simulink model "templateLCO"  (R2023a)
settings: Solver=VariableStepAuto  StartTime=0.0  StopTime=100  FixedStep=0.00001  MaxStep=0.001  RelTol=1e-5
undefined symbols (not defined in the file): A, B0, B1, B2, Ca, constantAeroForce, constantStruForce, D0, D1, D2, invMC, invMK, lref, Mhh, nAero, nStru, options, qInitial, rho, Ugap
libraries: cstblocks x1
settings Model: Creator=Nicola Fonzi  LastModifiedBy=nicol
settings SolverCC: ZeroCrossAlgorithm=Adaptive  AlgebraicLoopSolver=TrustRegion
settings DebuggingCC: UnconnectedInputMsg=warning  UnconnectedOutputMsg=warning  UnconnectedLineMsg=warning
settings ModelReferenceCC: EnableRefExpFcnMdlSchedulingChecks=on
settings RTWCC: DLArmComputeVersion=19.05

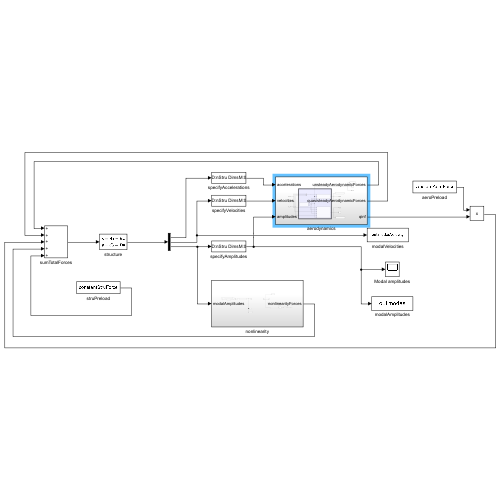
[thumbnail: Simulink's stored preview of the top-level diagram]
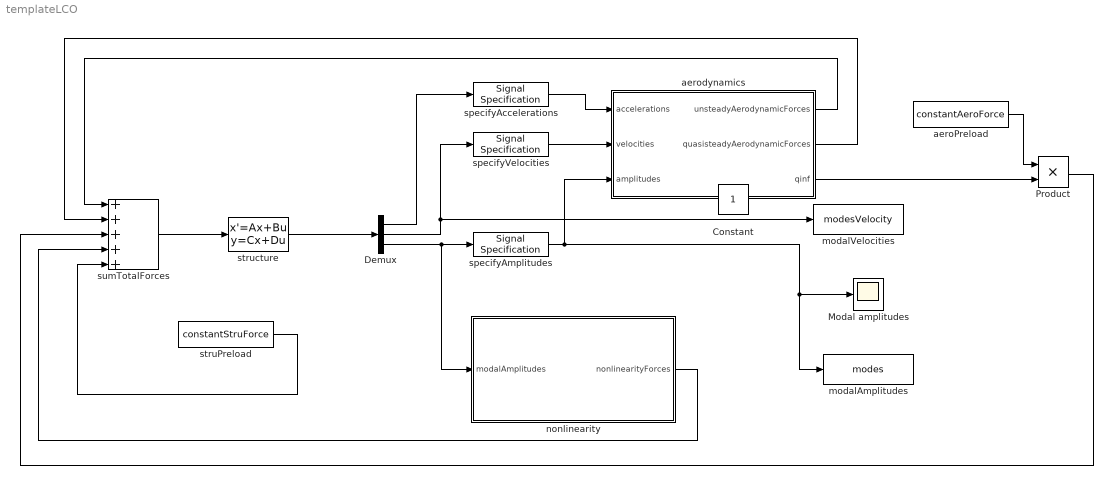
== system templateLCO ==
  Demux : Demux  Outputs=3
  Modal amplitudes : Scope
  Product : Product
  aeroPreload : Constant  Value=constantAeroForce
  aerodynamics : Subsystem
  modalAmplitudes : ToWorkspace  VariableName=modes  SaveFormat=Structure  SampleTime=-1
      settings: Save2DSignal=2-D array (concatenate along first dimension)
  modalVelocities : ToWorkspace  VariableName=modesVelocity  SaveFormat=Structure  SampleTime=-1
      settings: MaxDataPoints=1  Save2DSignal=2-D array (concatenate along first dimension)
  nonlinearity : Subsystem
  specifyAccelerations : SignalSpecification  Dimensions=nStru
  specifyAmplitudes : SignalSpecification  Dimensions=nStru
  specifyVelocities : SignalSpecification  Dimensions=nStru
  struPreload : Constant  Value=constantStruForce
  structure : StateSpace  A=[-invMC -invMK; eye(nStru) zeros(nStru)]  B=[inv(Mhh);zeros(nStru)]  C=[-invMC -invMK;eye(nStru) zeros(nStru);zeros(nStru) eye(nStru)]  D=[inv(Mhh);zeros(nStru);zeros(nStru)]  InitialCondition=qInitial
  sumTotalForces : Sum  Inputs=+++++
  Constant : Constant  IOType=siggen
  wires:
  structure/1 -> Demux/1
  sumTotalForces/1 -> structure/1
  Demux/3 -> nonlinearity/1(modalAmplitudes), specifyAmplitudes/1
  Demux/1 -> specifyAccelerations/1
  Demux/2 -> specifyVelocities/1, modalVelocities/1
  aerodynamics/1(unsteadyAerodynamicForces) -> sumTotalForces/1
  aerodynamics/2(quasisteadyAerodynamicForces) -> sumTotalForces/2
  specifyAccelerations/1 -> aerodynamics/1(accelerations)
  specifyVelocities/1 -> aerodynamics/2(velocities)
  specifyAmplitudes/1 -> modalAmplitudes/1, Modal amplitudes/1, aerodynamics/3(amplitudes)
  aerodynamics/3(qinf) -> Product/2
  aeroPreload/1 -> Product/1
  Product/1 -> sumTotalForces/3
  nonlinearity/1(nonlinearityForces) -> sumTotalForces/4
  struPreload/1 -> sumTotalForces/5

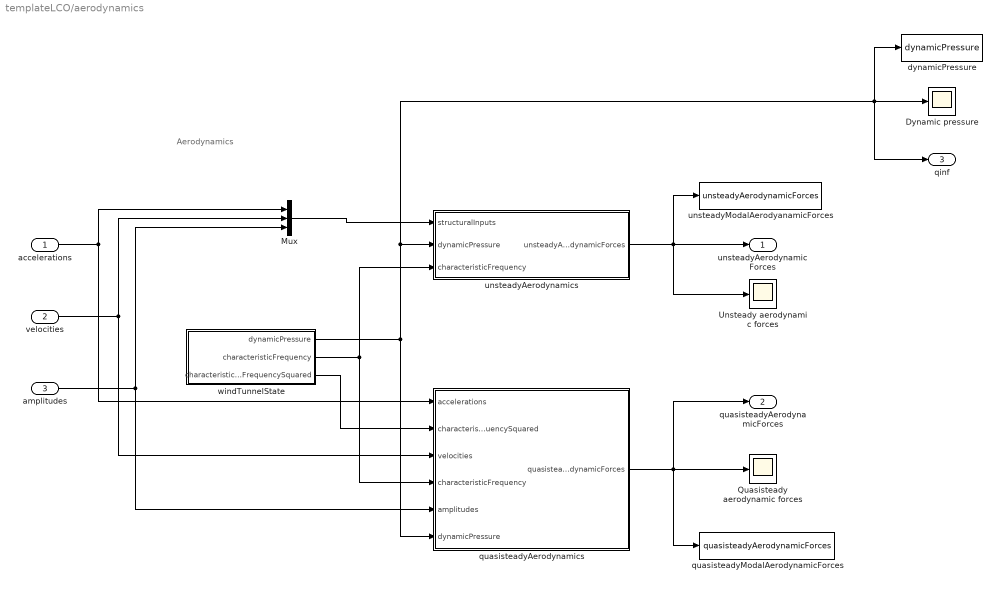
== system templateLCO/aerodynamics ==
  note: Aerodynamics
  accelerations : Inport
  velocities : Inport  Port=2
  amplitudes : Inport  Port=3
  Dynamic pressure : Scope
  Mux : Mux  Inputs=3
  Quasisteady aerodynamic forces : Scope
  Unsteady aerodynamic forces : Scope
  dynamicPressure : ToWorkspace  VariableName=dynamicPressure  SaveFormat=Structure  SampleTime=-1
      settings: Save2DSignal=2-D array (concatenate along first dimension)
  quasisteadyAerodynamics : Subsystem
  quasisteadyModalAerodynamicForces : ToWorkspace  VariableName=quasisteadyAerodynamicForces  SaveFormat=Structure  SampleTime=-1
      settings: Save2DSignal=2-D array (concatenate along first dimension)
  unsteadyAerodynamics : Subsystem
  unsteadyModalAerodyanamicForces : ToWorkspace  VariableName=unsteadyAerodynamicForces  SaveFormat=Structure  SampleTime=-1
      settings: Save2DSignal=2-D array (concatenate along first dimension)
  windTunnelState : Subsystem
  unsteadyAerodynamicForces : Outport
  quasisteadyAerodynamicForces : Outport  Port=2
  qinf : Outport  Port=3
  wires:
  windTunnelState/1(dynamicPressure) -> qinf/1, dynamicPressure/1, Dynamic pressure/1, unsteadyAerodynamics/2(dynamicPressure), quasisteadyAerodynamics/6(dynamicPressure)
  windTunnelState/2(characteristicFrequency) -> unsteadyAerodynamics/3(characteristicFrequency), quasisteadyAerodynamics/4(characteristicFrequency)
  windTunnelState/3(characteristicFrequencySquared) -> quasisteadyAerodynamics/2(characteristicFrequencySquared)
  accelerations/1 -> quasisteadyAerodynamics/1(accelerations), Mux/1
  velocities/1 -> quasisteadyAerodynamics/3(velocities), Mux/2
  amplitudes/1 -> quasisteadyAerodynamics/5(amplitudes), Mux/3
  Mux/1 -> unsteadyAerodynamics/1(structuralInputs)
  unsteadyAerodynamics/1(unsteadyAerodynamicForces) -> unsteadyModalAerodyanamicForces/1, Unsteady aerodynamic forces/1, unsteadyAerodynamicForces/1
  quasisteadyAerodynamics/1(quasisteadyAerodynamicForces) -> quasisteadyModalAerodynamicForces/1, quasisteadyAerodynamicForces/1, Quasisteady aerodynamic forces/1

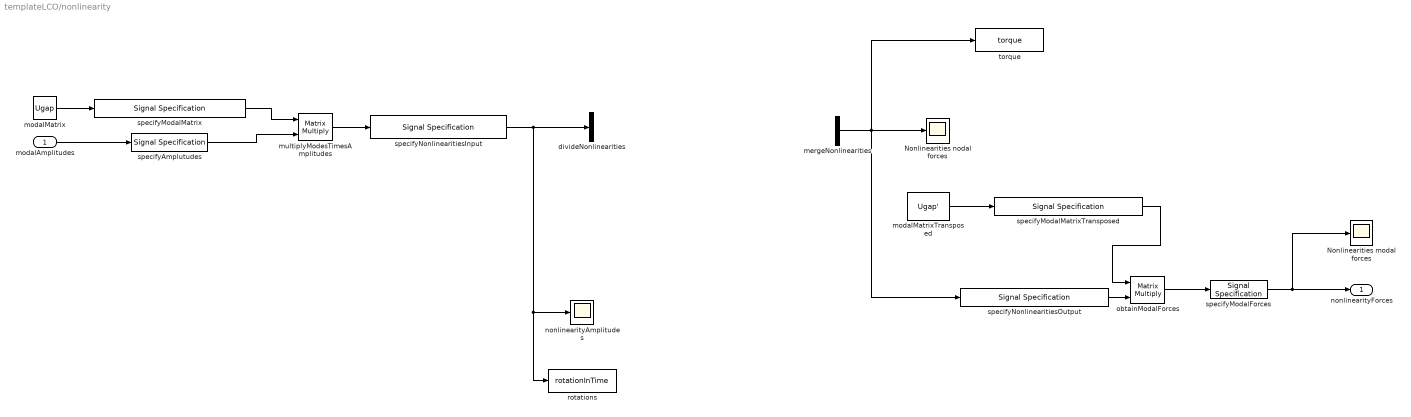
== system templateLCO/nonlinearity ==
  modalAmplitudes : Inport
  Nonlinearities modal forces : Scope
  Nonlinearities nodal forces : Scope
  divideNonlinearities : Demux  Outputs=2
  mergeNonlinearities : Mux  Inputs=2
  modalMatrix : Constant  Value=Ugap
  modalMatrixTransposed : Constant  Value=Ugap'
  multiplyModesTimesAmplitudes : Product  Multiplication=Matrix(*)
  nonlinearityAmplitudes : Scope
  obtainModalForces : Product  Multiplication=Matrix(*)
  rotations : ToWorkspace  VariableName=rotationInTime  SaveFormat=Structure With Time  SampleTime=-1
  specifyAmplutudes : SignalSpecification  Dimensions=[nStru,1]
  specifyModalForces : SignalSpecification  Dimensions=nStru
  specifyModalMatrix : SignalSpecification  Dimensions=[size(options.gapPoints,1),nStru]
  specifyModalMatrixTransposed : SignalSpecification  Dimensions=[nStru,size(options.gapPoints,1)]
  specifyNonlinearitiesInput : SignalSpecification  Dimensions=size(options.gapPoints,1)
  specifyNonlinearitiesOutput : SignalSpecification  Dimensions=[size(options.gapPoints,1),1]
  torque : ToWorkspace  VariableName=torque  SaveFormat=Structure With Time  SampleTime=-1
  nonlinearityForces : Outport
  wires:
  modalMatrixTransposed/1 -> specifyModalMatrixTransposed/1
  modalMatrix/1 -> specifyModalMatrix/1
  mergeNonlinearities/1 -> torque/1, specifyNonlinearitiesOutput/1, Nonlinearities nodal forces/1
  obtainModalForces/1 -> specifyModalForces/1
  specifyModalMatrix/1 -> multiplyModesTimesAmplitudes/1
  specifyAmplutudes/1 -> multiplyModesTimesAmplitudes/2
  modalAmplitudes/1 -> specifyAmplutudes/1
  specifyNonlinearitiesInput/1 -> divideNonlinearities/1, nonlinearityAmplitudes/1, rotations/1
  multiplyModesTimesAmplitudes/1 -> specifyNonlinearitiesInput/1
  specifyModalForces/1 -> nonlinearityForces/1, Nonlinearities modal forces/1
  specifyNonlinearitiesOutput/1 -> obtainModalForces/2
  specifyModalMatrixTransposed/1 -> obtainModalForces/1

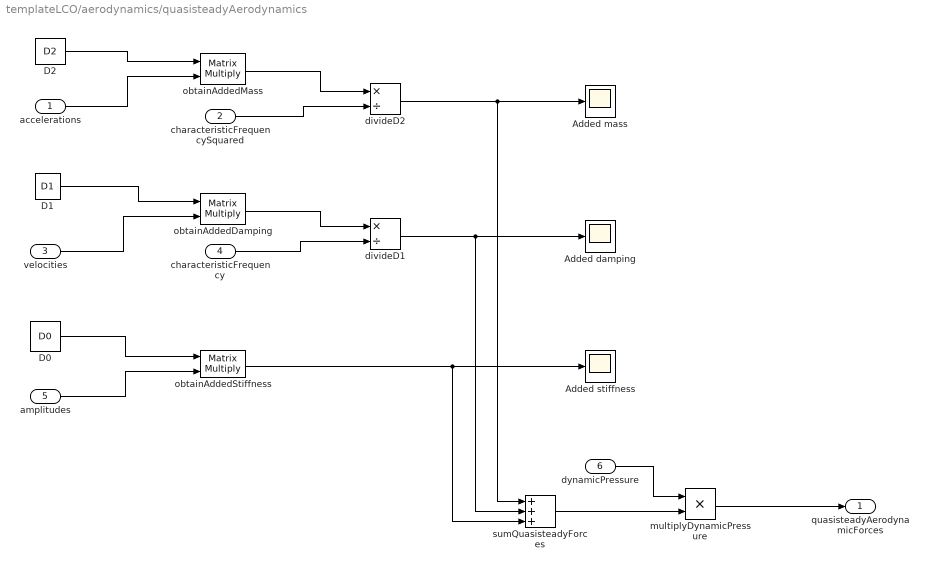
== system templateLCO/aerodynamics/quasisteadyAerodynamics ==
  accelerations : Inport
  characteristicFrequencySquared : Inport  Port=2
  velocities : Inport  Port=3
  characteristicFrequency : Inport  Port=4
  amplitudes : Inport  Port=5
  dynamicPressure : Inport  Port=6
  Added damping : Scope
  Added mass : Scope
  Added stiffness : Scope
  D0 : Constant  Value=D0
  D1 : Constant  Value=D1
  D2 : Constant  Value=D2
  divideD1 : Product  Inputs=*/
  divideD2 : Product  Inputs=*/
  multiplyDynamicPressure : Product
  obtainAddedDamping : Product  Multiplication=Matrix(*)
  obtainAddedMass : Product  Multiplication=Matrix(*)
  obtainAddedStiffness : Product  Multiplication=Matrix(*)
  sumQuasisteadyForces : Sum  Inputs=+++
  quasisteadyAerodynamicForces : Outport
  wires:
  amplitudes/1 -> obtainAddedStiffness/2
  obtainAddedDamping/1 -> divideD1/1
  divideD2/1 -> Added mass/1, sumQuasisteadyForces/1
  sumQuasisteadyForces/1 -> multiplyDynamicPressure/2
  dynamicPressure/1 -> multiplyDynamicPressure/1
  D2/1 -> obtainAddedMass/1
  divideD1/1 -> sumQuasisteadyForces/2, Added damping/1
  obtainAddedMass/1 -> divideD2/1
  D1/1 -> obtainAddedDamping/1
  obtainAddedStiffness/1 -> sumQuasisteadyForces/3, Added stiffness/1
  D0/1 -> obtainAddedStiffness/1
  velocities/1 -> obtainAddedDamping/2
  accelerations/1 -> obtainAddedMass/2
  characteristicFrequency/1 -> divideD1/2
  multiplyDynamicPressure/1 -> quasisteadyAerodynamicForces/1
  characteristicFrequencySquared/1 -> divideD2/2

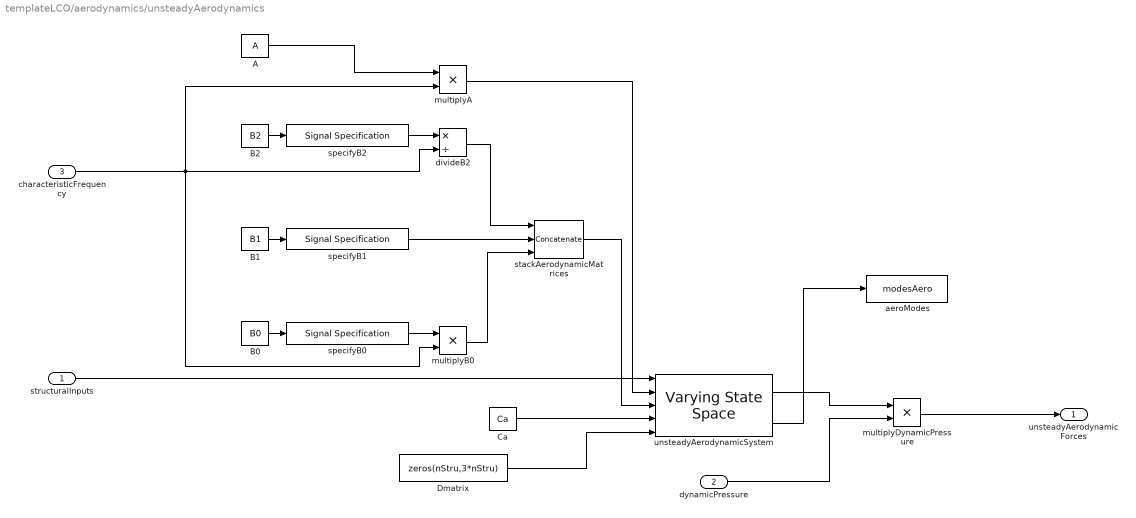
== system templateLCO/aerodynamics/unsteadyAerodynamics ==
  structuralInputs : Inport
  dynamicPressure : Inport  Port=2
  characteristicFrequency : Inport  Port=3
  A : Constant  Value=A
  B0 : Constant  Value=B0
  B1 : Constant  Value=B1
  B2 : Constant  Value=B2
  Ca : Constant  Value=Ca
  Dmatrix : Constant  Value=zeros(nStru,3*nStru)
  aeroModes : ToWorkspace  VariableName=modesAero  SaveFormat=Structure  SampleTime=-1
      settings: MaxDataPoints=1  Save2DSignal=2-D array (concatenate along first dimension)
  divideB2 : Product  Inputs=*/
  multiplyA : Product  Inputs=**
  multiplyB0 : Product  Inputs=**
  multiplyDynamicPressure : Product
  specifyB0 : SignalSpecification  Dimensions=[nAero,nStru]
  specifyB1 : SignalSpecification  Dimensions=[nAero,nStru]
  specifyB2 : SignalSpecification  Dimensions=[nAero,nStru]
  stackAerodynamicMatrices : Concatenate  NumInputs=3  Mode=Multidimensional array  ConcatenateDimension=2
  unsteadyAerodynamicSystem : cstblocks/Linear Parameter Varying/Varying State Space  x0=qInitialAero  xNames=''  OutputX=on  OutputDX=off
  unsteadyAerodynamicForces : Outport
  wires:
  multiplyA/1 -> unsteadyAerodynamicSystem/2
  characteristicFrequency/1 -> multiplyA/2, divideB2/2, multiplyB0/2
  A/1 -> multiplyA/1
  B1/1 -> specifyB1/1
  unsteadyAerodynamicSystem/1 -> multiplyDynamicPressure/1
  divideB2/1 -> stackAerodynamicMatrices/1
  B0/1 -> specifyB0/1
  Ca/1 -> unsteadyAerodynamicSystem/4
  B2/1 -> specifyB2/1
  stackAerodynamicMatrices/1 -> unsteadyAerodynamicSystem/3
  multiplyB0/1 -> stackAerodynamicMatrices/3
  Dmatrix/1 -> unsteadyAerodynamicSystem/5
  dynamicPressure/1 -> multiplyDynamicPressure/2
  structuralInputs/1 -> unsteadyAerodynamicSystem/1
  multiplyDynamicPressure/1 -> unsteadyAerodynamicForces/1
  specifyB2/1 -> divideB2/1
  specifyB1/1 -> stackAerodynamicMatrices/2
  specifyB0/1 -> multiplyB0/1
  unsteadyAerodynamicSystem/2 -> aeroModes/1

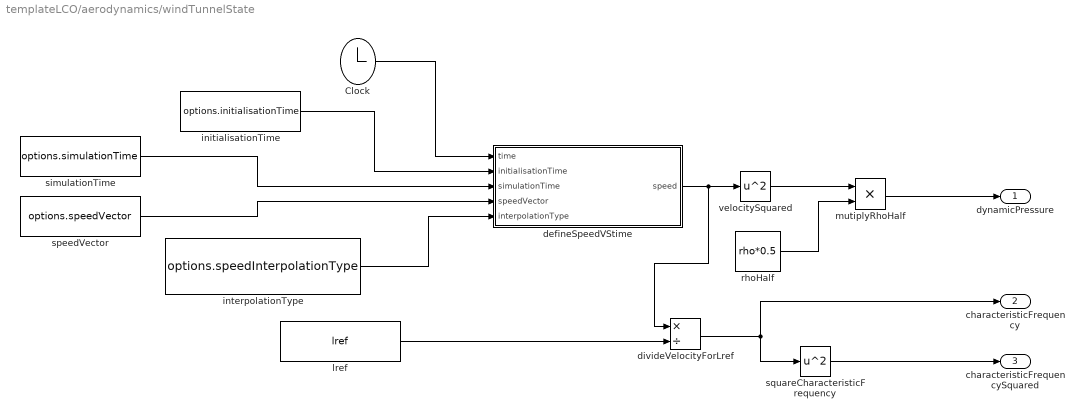
== system templateLCO/aerodynamics/windTunnelState ==
  Clock : Clock
  defineSpeedVStime : MATLAB Function  TreatAsAtomicUnit=on
  divideVelocityForLref : Product  Inputs=*/
  initialisationTime : Constant  Value=options.initialisationTime
  interpolationType : Constant  Value=options.speedInterpolationType
  lref : Constant  Value=lref
  mutiplyRhoHalf : Product
  rhoHalf : Constant  Value=rho*0.5
  simulationTime : Constant  Value=options.simulationTime
  speedVector : Constant  Value=options.speedVector
  squareCharacteristicFrequency : Math  Operator=square
  velocitySquared : Math  Operator=square
  dynamicPressure : Outport
  characteristicFrequency : Outport  Port=2
  characteristicFrequencySquared : Outport  Port=3
  wires:
  divideVelocityForLref/1 -> characteristicFrequency/1, squareCharacteristicFrequency/1
  Clock/1 -> defineSpeedVStime/1(time)
  lref/1 -> divideVelocityForLref/2
  defineSpeedVStime/1(speed) -> velocitySquared/1, divideVelocityForLref/1
  velocitySquared/1 -> mutiplyRhoHalf/1
  rhoHalf/1 -> mutiplyRhoHalf/2
  mutiplyRhoHalf/1 -> dynamicPressure/1
  squareCharacteristicFrequency/1 -> characteristicFrequencySquared/1
  initialisationTime/1 -> defineSpeedVStime/2(initialisationTime)
  speedVector/1 -> defineSpeedVStime/4(speedVector)
  simulationTime/1 -> defineSpeedVStime/3(simulationTime)
  interpolationType/1 -> defineSpeedVStime/5(interpolationType)

== matlab function templateLCO/aerodynamics/windTunnelState/defineSpeedVStime ==
  data: time input; speed output; initialisationTime input; simulationTime input; speedVector input; interpolationType input
function speed = fcn(time,initialisationTime,simulationTime,speedVector,interpolationType  )


if time<=initialisationTime || length(speedVector)==1
    speed = speedVector(1);
else
    if interpolationType==0
        speed = interp1(linspace(initialisationTime,simulationTime...
            ,length(speedVector)+1),[speedVector; speedVector(end)],time,'previous');
    elseif interpolationType==1
        speed = interp1(linspace(initialisationTime,simulationTime,length(speedVector))...
            ,speedVector,time,'linear');
    else
        speed = interp1(linspace(initialisationTime,simulationTime,length(speedVector))...
            ,speedVector,time,'spline');
    end
end

return
